simulink model "Test_model_671203"  (R2024a)
settings: Solver=VariableStepAuto  StartTime=0.0  StopTime=10  RelTol=1e-3
undefined symbols (not defined in the file or in its folder): X, Y, Z
libraries: sm_lib x63, nesl_utility x21
(part 1 of 3)
settings Model: Creator=pimna  LastModifiedBy=pimna

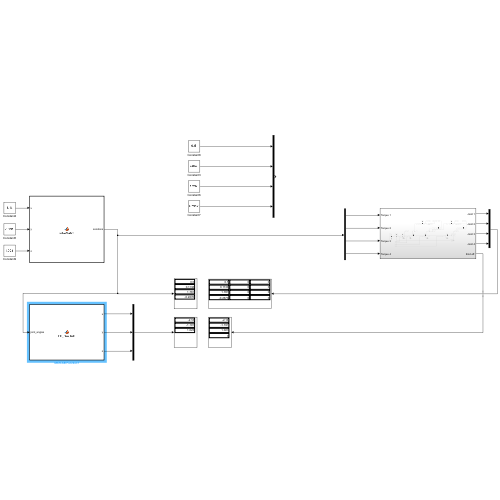
[thumbnail: Simulink's stored preview of the top-level diagram]
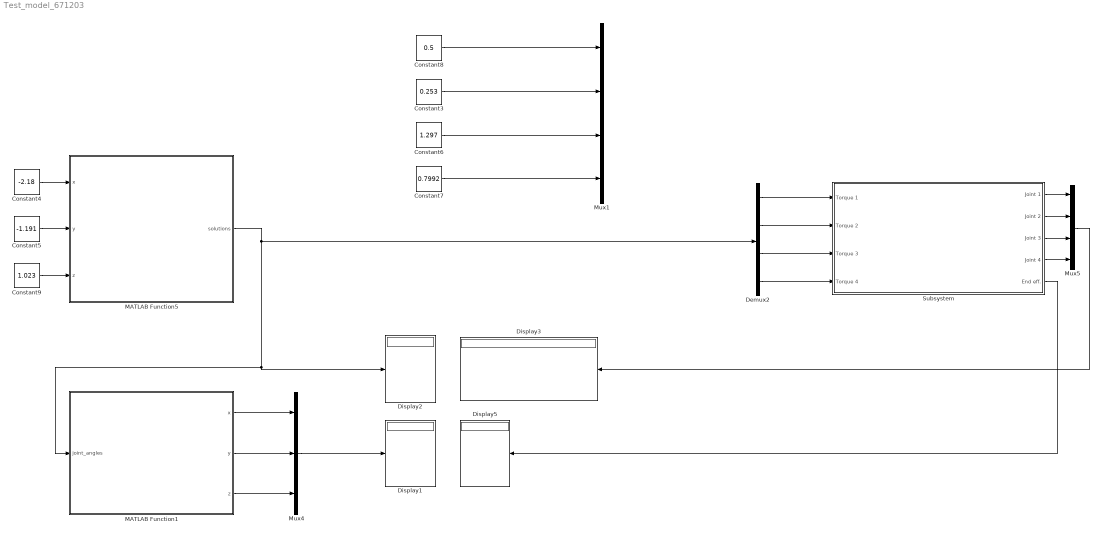
== system Test_model_671203 ==
  Constant3 : Constant  Value=0.253  VectorParams1D=off  SampleTime=-1
  Constant4 : Constant  Value=-2.18  SampleTime=-1
  Constant5 : Constant  Value=-1.191  SampleTime=-1
  Constant6 : Constant  Value=1.297  VectorParams1D=off  SampleTime=-1
  Constant7 : Constant  Value=0.7992  VectorParams1D=off  SampleTime=-1
  Constant8 : Constant  Value=0.5  VectorParams1D=off  SampleTime=-1
  Constant9 : Constant  Value=1.023  SampleTime=-1
  Demux2 : Demux
  Display{1..3,5} (4 alike) : Display
  MATLAB Function1 : MATLAB Function  TreatAsAtomicUnit=on
  MATLAB Function5 : MATLAB Function  TreatAsAtomicUnit=on
  Mux1 : Mux
  Mux4 : Mux  Inputs=3
  Mux5 : Mux
  Subsystem : Subsystem
  wires:
  Subsystem/1(Joint 1) -> Mux5/1
  Subsystem/2(Joint 2) -> Mux5/2
  Subsystem/3(Joint 3) -> Mux5/3
  Subsystem/4(Joint 4) -> Mux5/4
  Mux5/1 -> Display3/1
  Subsystem/5(End eff.) -> Display5/1
  Constant9/1 -> MATLAB Function5/3(z)
  Constant4/1 -> MATLAB Function5/1(x)
  Constant5/1 -> MATLAB Function5/2(y)
  MATLAB Function5/1(solutions) -> Demux2/1, MATLAB Function1/1(joint_angles), Display2/1
  MATLAB Function1/3(z) -> Mux4/3
  MATLAB Function1/2(y) -> Mux4/2
  Mux4/1 -> Display1/1
  MATLAB Function1/1(x) -> Mux4/1
  Demux2/1 -> Subsystem/1(Torque 1)
  Demux2/2 -> Subsystem/2(Torque 2)
  Demux2/3 -> Subsystem/3(Torque 3)
  Demux2/4 -> Subsystem/4(Torque 4)
  Constant6/1 -> Mux1/3
  Constant7/1 -> Mux1/4
  Constant3/1 -> Mux1/2
  Constant8/1 -> Mux1/1
